simulink model "ReferenceModel"  (R2024a)
settings: Solver=VariableStepAuto  StartTime=0.0  StopTime=10.0  RelTol=1e-3
values from neighbouring files (symbols this model uses):
  A = [0 1 0; 0 0 1; 0 -g/l 0]    [EENG417_p2fromAidhen.m]    (also in LandKDet.m)
  B = [0; 0; 1]    [EENG417_p2fromAidhen.m]    (also in LandKDet.m)
  C = [g/l 0 0]    [EENG417_p2fromAidhen.m]    (also in LandKDet.m)
  K = place(A,B, Poles_K)    [EENG417_p2fromAidhen.m]    (also in LandKDet.m)
  L = place(A',C', Poles_L).'    [EENG417_p2fromAidhen.m]    (also in LandKDet.m = place(A',C', Poles_L)')
  N = -1/(C*((A-B*K)\B))    [EENG417_p2fromAidhen.m]    (also in LandKDet.m = 1 / (C * inv(-A + B*K) * B))
settings Model: Creator=Aidhen  LastModifiedBy=Aidhen

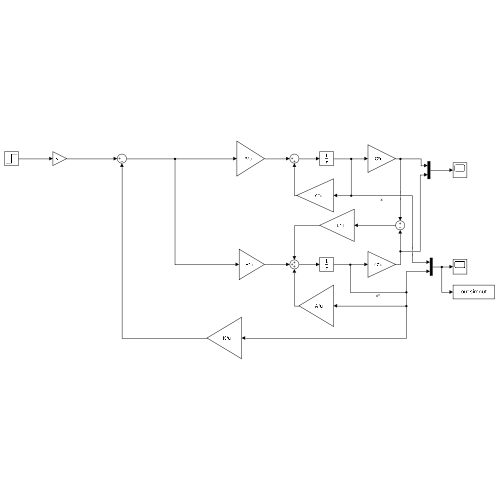
[thumbnail: Simulink's stored preview of the top-level diagram]
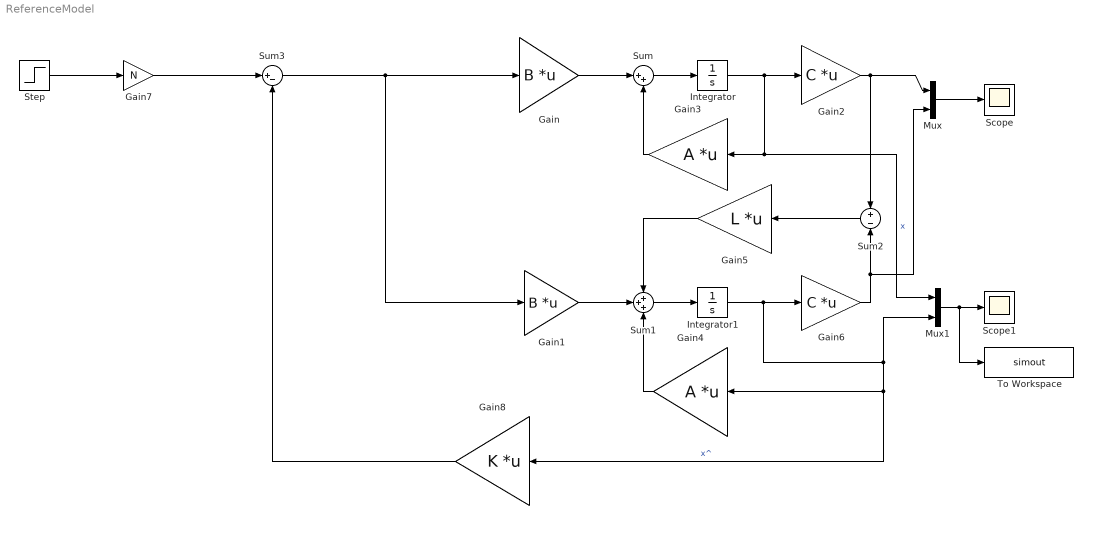
== system ReferenceModel ==
  Gain : Gain  Gain=B  Multiplication=Matrix(K*u)
  Gain1 : Gain  Gain=B  Multiplication=Matrix(K*u)
  Gain2 : Gain  Gain=C  Multiplication=Matrix(K*u)
  Gain3 : Gain  Gain=A  Multiplication=Matrix(K*u)
  Gain4 : Gain  Gain=A  Multiplication=Matrix(K*u)
  Gain5 : Gain  Gain=L  Multiplication=Matrix(K*u)
  Gain6 : Gain  Gain=C  Multiplication=Matrix(K*u)
  Gain7 : Gain  Gain=N
  Gain8 : Gain  Gain=K  Multiplication=Matrix(K*u)
  Integrator : Integrator  InitialCondition=[1 ;1;1]
  Integrator1 : Integrator  InitialCondition=[0;0;0]
  Mux : Mux  Inputs=2
  Mux1 : Mux  Inputs=2
  Scope : Scope
  Scope1 : Scope
  Step : Step  SampleTime=0
  Sum : Sum  Inputs=|++
  Sum1 : Sum  Inputs=+++
  Sum2 : Sum  Inputs=+-
  Sum3 : Sum  Inputs=|+-
  To Workspace : ToWorkspace  VariableName=simout  SaveFormat=Timeseries  SampleTime=-1
  wires:
  Mux1/1 -> To Workspace/1, Scope1/1
  Mux/1 -> Scope/1
  Sum2/1 -> Gain5/1
  Gain2/1 -> Sum2/1, Mux/1
  Gain5/1 -> Sum1/1
  Sum/1 -> Integrator/1
  Gain6/1 -> Mux/2, Sum2/2
  Gain1/1 -> Sum1/2
  Integrator/1 -> Mux1/1, Gain3/1, Gain2/1  "x"
  Integrator1/1 -> Gain6/1, Mux1/2, Gain8/1, Gain4/1  "x^"
  Sum1/1 -> Integrator1/1
  Gain4/1 -> Sum1/3
  Gain/1 -> Sum/1
  Gain3/1 -> Sum/2
  Gain7/1 -> Sum3/1
  Sum3/1 -> Gain1/1, Gain/1
  Gain8/1 -> Sum3/2
  Step/1 -> Gain7/1
